simulink model "robot_reglage"  (R2017a)
settings: Solver=VariableStepAuto  StartTime=0.0  StopTime=10.0  RelTol=1e-3
values from neighbouring files (symbols this model uses):
  F1 = 30    [robot.m]
  k1 = 100    [robot.m]
  Kd = 2    [robot.m]
  Kp = 2    [robot.m]
  m1 = 10    [robot.m]
  m2 = 5    [robot.m]
  m3 = 5    [robot.m]
settings Model: Creator=massona  LastModifiedBy=massona
settings DataIOCC: Refine=100

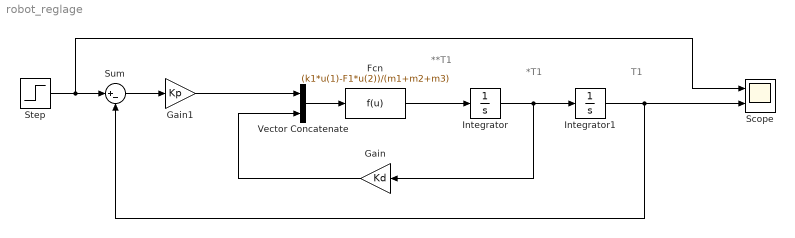
== system robot_reglage ==
  note: **T1
  note: *T1
  note: T1
  Fcn : Fcn  Expr=(k1*u(1)-F1*u(2))/(m1+m2+m3)
  Gain : Gain  Gain=Kd
  Gain1 : Gain  Gain=Kp
  Integrator : Integrator
  Integrator1 : Integrator
  Scope : Scope  NumInputPorts=2
  Step : Step  SampleTime=0
  Sum : Sum  Inputs=|+-
  Vector Concatenate : Concatenate
  wires:
  Vector Concatenate/1 -> Fcn/1
  Fcn/1 -> Integrator/1
  Integrator/1 -> Integrator1/1, Gain/1
  Gain/1 -> Vector Concatenate/2
  Gain1/1 -> Vector Concatenate/1
  Sum/1 -> Gain1/1
  Integrator1/1 -> Scope/2, Sum/2
  Step/1 -> Scope/1, Sum/1
